simulink model "hwTarget"  (R2020b)
settings: Solver=VariableStepAuto  StartTime=0.0  StopTime=Ts  RelTol=1e-3
InitFcn:
  | evalin('base','pixelcontrolbus');
  | 
  | ROWS = 480;
  | COLS = 752;
  | 
  | OFFSET = 3;
  | imagesToRead = 20;
  | Ts = (imagesToRead + OFFSET) * 2;
  | 
  | inputNums = [1:imagesToRead];
  | 
  | MagThrL = 7;
  | MagThrS = 3;
  | SegMaxLength = 630;
  | 
  | NUM_OF_BITS = 32;
  | MSB = NUM_OF_BITS-1;
  | cap_1 = fixdt(0,NUM_OF_BITS,NUM_OF_BITS-1);
  | cap_2 = fixdt(0,NUM_OF_BITS,NUM_OF_BITS-2);
  | 
  | CORDIC_LUT_DT_1 = fixdt(1, NUM_OF_BITS, NUM_OF_BITS-2);
  | CORDIC_LUT_DT_2 = fixdt(1, NUM_OF_BITS, NUM_OF_BITS-1);
  | CORDIC_LUT_DT_3 = fixdt(1, NUM_OF_BITS, NUM_OF_BITS);
  | CORDIC_LUT_DT_4 = fixdt(1, NUM_OF_BITS, NUM_OF_BITS+1);
  | CORDIC_LUT_DT_5 = fixdt(1, NUM_OF_BITS, NUM_OF_BITS+1);
  | CORDIC_LUT_DT_6 = fixdt(1, NUM_OF_BITS, NUM_OF_BITS+2);
  | CORDIC_LUT_DT_7 = fixdt(1, NUM_OF_BITS, NUM_OF_BITS+3);
  | CORDIC_LUT_DT_8 = fixdt(1, NUM_OF_BITS, NUM_OF_BITS+4);
  | CORDIC_LUT_DT_9 = fixdt(1, NUM_OF_BITS, NUM_OF_BITS+5);
  | CORDIC_LUT_DT_10 = fixdt(1, NUM_OF_BITS, NUM_OF_BITS+6);
  | CORDIC_LUT_DT_11 = fixdt(1, NUM_OF_BITS, NUM_OF_BITS+7);
  | CORDIC_LUT_DT_12 = fixdt(1, NUM_OF_BITS, NUM_OF_BITS+8);
  | 
  | RGB_DT = fixdt(0, 24, 0);
  | GRAY_DT = fixdt(0, 8, 0);
  | THETA_DT = fixdt(1, 16, 13);
  | MAG_DT = fixdt(0, 16, 15);
  | KIRCH_DT = fixdt(0, 12, 0);
undefined symbols (not defined in the file or in its folder): bufferInit, bufferSize
libraries: hdlsllib x86, simulink x6, visionhdlstatistics x4, visionhdlio x2, visionhdlutilities x1
(part 3 of 3)

== system hwTarget/hwTarget/Kirsch Operation Northwest/Kirch Filter North-West/Kirch Filter/slicer ==
  note: 5 | 5 |-3
      | 5 | 0 |-3
      | -3 |-3 |-3
  data_in : Inport
  Delay{1..6} (6 alike) : Delay  DelayLength=1  InitialCondition=0
  Display : Display
  Display1 : Display
  Line buffer : Delay  DelayLength=COLS-2  InitialCondition=0
  Line buffer1 : Delay  DelayLength=COLS-2  InitialCondition=0
  Mux : Mux  Inputs=3
  Mux1 : Mux  Inputs=5
  Fives : Outport
  nThrees : Outport  Port=2
  wires:
  Delay4/1 -> Mux1/3, Line buffer/1
  data_in/1 -> Mux1/5, Delay1/1
  Delay1/1 -> Mux1/4, Delay4/1
  Delay3/1 -> Mux/2, Delay6/1
  Delay5/1 -> Line buffer1/1, Mux/3
  Line buffer/1 -> Mux1/2, Delay2/1
  Line buffer1/1 -> Delay3/1, Mux1/1
  Delay2/1 -> Delay5/1
  Mux/1 -> Display1/1, Fives/1
  Mux1/1 -> Display/1, nThrees/1
  Delay6/1 -> Mux/1

== system hwTarget/hwTarget/Kirsch Operation Southwest/Binarize/Subsystem/MagThrL ==
  mean : Inport
  stddev : Inport  Port=2
  dev_step : Inport  Port=3
  Add1 : Sum
  Product : Product
  thresh : Outport
  wires:
  stddev/1 -> Product/1
  mean/1 -> Add1/1
  dev_step/1 -> Product/2
  Product/1 -> Add1/2
  Add1/1 -> thresh/1

== system hwTarget/hwTarget/Kirsch Operation Southwest/Binarize/Subsystem/MagThrS ==
  mean : Inport
  stddev : Inport  Port=2
  dev_step : Inport  Port=3
  Add1 : Sum
  Product : Product
  thresh : Outport
  wires:
  stddev/1 -> Product/1
  mean/1 -> Add1/1
  dev_step/1 -> Product/2
  Product/1 -> Add1/2
  Add1/1 -> thresh/1

== system hwTarget/hwTarget/Kirsch Operation Southwest/Kirch Filter South-West/Subsystem/slicer ==
  note: -3 |-3 |-3
      | 5 | 0 |-3
      | 5 | 5 |-3
  data_in : Inport
  Delay{1..6} (6 alike) : Delay  DelayLength=1  InitialCondition=0
  Display : Display
  Display1 : Display
  Line buffer : Delay  DelayLength=COLS-2  InitialCondition=0
  Line buffer1 : Delay  DelayLength=COLS-2  InitialCondition=0
  Mux : Mux  Inputs=3
  Mux1 : Mux  Inputs=5
  Fives : Outport
  nThrees : Outport  Port=2
  wires:
  Delay4/1 -> Line buffer/1, Mux/2
  data_in/1 -> Mux1/5, Delay1/1
  Delay1/1 -> Mux/3, Delay4/1
  Delay3/1 -> Mux1/2, Delay6/1
  Delay5/1 -> Line buffer1/1, Mux/1
  Line buffer/1 -> Mux1/4, Delay2/1
  Line buffer1/1 -> Mux1/3, Delay3/1
  Delay2/1 -> Delay5/1
  Mux/1 -> Display1/1, Fives/1
  Mux1/1 -> Display/1, nThrees/1
  Delay6/1 -> Mux1/1

== system hwTarget/hwTarget/Kirsch Operation West/Binarize/Subsystem/MagThrL ==
  mean : Inport
  stddev : Inport  Port=2
  dev_step : Inport  Port=3
  Add1 : Sum
  Product : Product
  thresh : Outport
  wires:
  stddev/1 -> Product/1
  mean/1 -> Add1/1
  dev_step/1 -> Product/2
  Product/1 -> Add1/2
  Add1/1 -> thresh/1

== system hwTarget/hwTarget/Kirsch Operation West/Binarize/Subsystem/MagThrS ==
  mean : Inport
  stddev : Inport  Port=2
  dev_step : Inport  Port=3
  Add1 : Sum
  Product : Product
  thresh : Outport
  wires:
  stddev/1 -> Product/1
  mean/1 -> Add1/1
  dev_step/1 -> Product/2
  Product/1 -> Add1/2
  Add1/1 -> thresh/1

== system hwTarget/hwTarget/Kirsch Operation West/Kirch Filter West/Subsystem/slicer ==
  note: 5 |-3 |-3
      | 5 | 0 |-3
      | 5 |-3 |-3
  data_in : Inport
  Delay{1..6} (6 alike) : Delay  DelayLength=1  InitialCondition=0
  Display : Display
  Display1 : Display
  Line buffer : Delay  DelayLength=COLS-2  InitialCondition=0
  Line buffer1 : Delay  DelayLength=COLS-2  InitialCondition=0
  Mux : Mux  Inputs=3
  Mux1 : Mux  Inputs=5
  Fives : Outport
  nThrees : Outport  Port=2
  wires:
  Delay4/1 -> Mux/3, Line buffer/1
  data_in/1 -> Mux1/5, Delay1/1
  Delay1/1 -> Mux1/4, Delay4/1
  Delay3/1 -> Mux1/1, Delay6/1
  Delay5/1 -> Mux/2, Line buffer1/1
  Line buffer/1 -> Mux1/3, Delay2/1
  Line buffer1/1 -> Mux1/2, Delay3/1
  Delay2/1 -> Delay5/1
  Mux/1 -> Display1/1, Fives/1
  Mux1/1 -> Display/1, nThrees/1
  Delay6/1 -> Mux/1

== system hwTarget/hwTarget/Segmentation/North Segmentation/Enabled Subsystem1/Enabled Subsystem ==
  In1 : Inport
  Enable : EnablePort
  To Workspace7 : ToWorkspace  VariableName=officialResults  SaveFormat=Timeseries  SampleTime=-1
  wires:
  In1/1 -> To Workspace7/1

== system hwTarget/hwTarget/Segmentation/North Segmentation/Enabled Subsystem1/Subsystem ==
  u : Inport
  Bit Slice : hdlsllib/Logic and Bit Operations/Bit Slice  lidx=47  ridx=32
      settings: SourceProductBaseCode=SL
  Bit Slice1 : hdlsllib/Logic and Bit Operations/Bit Slice  lidx=31  ridx=16
      settings: SourceProductBaseCode=SL
  Bit Slice2 : hdlsllib/Logic and Bit Operations/Bit Slice  lidx=15  ridx=0
      settings: SourceProductBaseCode=SL
  x : Outport
  y : Outport  Port=2
  theta : Outport  Port=3
  wires:
  u/1 -> Bit Slice2/1, Bit Slice1/1, Bit Slice/1
  Bit Slice2/1 -> theta/1
  Bit Slice/1 -> x/1
  Bit Slice1/1 -> y/1

== system hwTarget/hwTarget/Segmentation/North Segmentation/Enabled Subsystem1/Subsystem1 ==
  u : Inport
  Bit Slice : hdlsllib/Logic and Bit Operations/Bit Slice  lidx=47  ridx=32
      settings: SourceProductBaseCode=SL
  Bit Slice1 : hdlsllib/Logic and Bit Operations/Bit Slice  lidx=31  ridx=16
      settings: SourceProductBaseCode=SL
  Bit Slice2 : hdlsllib/Logic and Bit Operations/Bit Slice  lidx=15  ridx=0
      settings: SourceProductBaseCode=SL
  x : Outport
  y : Outport  Port=2
  theta : Outport  Port=3
  wires:
  Bit Slice1/1 -> y/1
  Bit Slice/1 -> x/1
  Bit Slice2/1 -> theta/1
  u/1 -> Bit Slice/1, Bit Slice1/1, Bit Slice2/1

== system hwTarget/hwTarget/Segmentation/North Segmentation/Enabled Subsystem1/Subsystem2 ==
  u : Inport
  Bit Slice : hdlsllib/Logic and Bit Operations/Bit Slice  lidx=47  ridx=32
      settings: SourceProductBaseCode=SL
  Bit Slice1 : hdlsllib/Logic and Bit Operations/Bit Slice  lidx=31  ridx=16
      settings: SourceProductBaseCode=SL
  Bit Slice2 : hdlsllib/Logic and Bit Operations/Bit Slice  lidx=15  ridx=0
      settings: SourceProductBaseCode=SL
  x : Outport
  y : Outport  Port=2
  theta : Outport  Port=3
  wires:
  u/1 -> Bit Slice2/1, Bit Slice1/1, Bit Slice/1
  Bit Slice2/1 -> theta/1
  Bit Slice/1 -> x/1
  Bit Slice1/1 -> y/1

== system hwTarget/hwTarget/Segmentation/North Segmentation/Enabled Subsystem1/Subsystem3 ==
  u : Inport
  Bit Slice : hdlsllib/Logic and Bit Operations/Bit Slice  lidx=47  ridx=32
      settings: SourceProductBaseCode=SL
  Bit Slice1 : hdlsllib/Logic and Bit Operations/Bit Slice  lidx=31  ridx=16
      settings: SourceProductBaseCode=SL
  Bit Slice2 : hdlsllib/Logic and Bit Operations/Bit Slice  lidx=15  ridx=0
      settings: SourceProductBaseCode=SL
  x : Outport
  y : Outport  Port=2
  theta : Outport  Port=3
  wires:
  Bit Slice1/1 -> y/1
  Bit Slice/1 -> x/1
  Bit Slice2/1 -> theta/1
  u/1 -> Bit Slice/1, Bit Slice1/1, Bit Slice2/1

== system hwTarget/hwTarget/Segmentation/North Segmentation/minXReadSwitch/Subsystem1 ==
  reset : Inport
  Constant : Constant  OutDataTypeStr=fixdt(0,10,0)  SampleTime=-1
  Delay2 : Delay  DelayLength=1  InitialCondition=0  ExternalReset=Level
      settings: InputPortMap=u0,r5
  Sum : Sum  Inputs=|++  OutDataTypeStr=uint16
  counter : Outport
  wires:
  reset/1 -> Delay2/2
  Delay2/1 -> Sum/1
  Constant/1 -> Sum/2
  Sum/1 -> Delay2/1, counter/1  "blobID"

== system hwTarget/hwTarget/Segmentation/North Segmentation/minXReadSwitch1/Subsystem1 ==
  reset : Inport
  Constant : Constant  OutDataTypeStr=fixdt(0,10,0)  SampleTime=-1
  Delay2 : Delay  DelayLength=1  InitialCondition=0  ExternalReset=Level
      settings: InputPortMap=u0,r5
  Sum : Sum  Inputs=|++  OutDataTypeStr=uint16
  counter : Outport
  wires:
  reset/1 -> Delay2/2
  Delay2/1 -> Sum/1
  Constant/1 -> Sum/2
  Sum/1 -> Delay2/1, counter/1  "blobID"

== system hwTarget/hwTarget/Segmentation/North Segmentation/minXReadSwitch3/Subsystem1 ==
  reset : Inport
  Constant : Constant  OutDataTypeStr=fixdt(0,10,0)  SampleTime=-1
  Delay2 : Delay  DelayLength=1  InitialCondition=0  ExternalReset=Level
      settings: InputPortMap=u0,r5
  Sum : Sum  Inputs=|++  OutDataTypeStr=uint16
  counter : Outport
  wires:
  reset/1 -> Delay2/2
  Delay2/1 -> Sum/1
  Constant/1 -> Sum/2
  Sum/1 -> Delay2/1, counter/1  "blobID"

== system hwTarget/hwTarget/Segmentation/North Segmentation/minXSwitch4/Subsystem ==
  reset : Inport
  Constant : Constant  OutDataTypeStr=fixdt(0,10,0)  SampleTime=-1
  Delay2 : Delay  DelayLength=1  InitialCondition=0  ExternalReset=Level
      settings: InputPortMap=u0,r5
  Sum : Sum  Inputs=|++  OutDataTypeStr=uint16
  counter : Outport
  wires:
  Sum/1 -> counter/1, Delay2/1  "blobID"
  Constant/1 -> Sum/2
  Delay2/1 -> Sum/1
  reset/1 -> Delay2/2

== system hwTarget/hwTarget/Segmentation/North Segmentation/minXSwitch4/Subsystem1 ==
  reset : Inport
  Constant : Constant  OutDataTypeStr=fixdt(0,10,0)  SampleTime=-1
  Delay2 : Delay  DelayLength=1  InitialCondition=0  ExternalReset=Level
      settings: InputPortMap=u0,r5
  Sum : Sum  Inputs=|++  OutDataTypeStr=uint16
  counter : Outport
  wires:
  reset/1 -> Delay2/2
  Delay2/1 -> Sum/1
  Constant/1 -> Sum/2
  Sum/1 -> Delay2/1, counter/1  "blobID"

== system hwTarget/hwTarget/CordicAtan/CORDIC Algorithm/Iteration_10/X_Logic/zsign ==
  signof : Inport
  base : Inport  Port=2
  Bit Slice : hdlsllib/Logic and Bit Operations/Bit Slice  lidx=MSB  ridx=MSB
      settings: SourceProductBaseCode=SL
  Switch : Switch  Criteria=u2 > Threshold
  Unary Minus : UnaryMinus
  out : Outport
  wires:
  signof/1 -> Bit Slice/1
  Bit Slice/1 -> Switch/2
  base/1 -> Switch/3, Unary Minus/1
  Switch/1 -> out/1
  Unary Minus/1 -> Switch/1

== system hwTarget/hwTarget/CordicAtan/CORDIC Algorithm/Iteration_10/Y_Logic/n_zsign ==
  signof : Inport
  base : Inport  Port=2
  Bit Slice : hdlsllib/Logic and Bit Operations/Bit Slice  lidx=MSB  ridx=MSB
      settings: SourceProductBaseCode=SL
  Switch : Switch  Criteria=u2 > Threshold
  Unary Minus : UnaryMinus
  out : Outport
  wires:
  Bit Slice/1 -> Switch/2
  signof/1 -> Bit Slice/1
  base/1 -> Switch/1, Unary Minus/1
  Switch/1 -> out/1
  Unary Minus/1 -> Switch/3

== system hwTarget/hwTarget/CordicAtan/CORDIC Algorithm/Iteration_2/X_Logic/zsign1 ==
  signof : Inport
  base : Inport  Port=2
  Bit Slice : hdlsllib/Logic and Bit Operations/Bit Slice  lidx=MSB  ridx=MSB
      settings: SourceProductBaseCode=SL
  Switch : Switch  Criteria=u2 > Threshold
  Unary Minus : UnaryMinus
  out : Outport
  wires:
  signof/1 -> Bit Slice/1
  Bit Slice/1 -> Switch/2
  base/1 -> Switch/3, Unary Minus/1
  Switch/1 -> out/1
  Unary Minus/1 -> Switch/1

== system hwTarget/hwTarget/CordicAtan/CORDIC Algorithm/Iteration_2/Y_Logic/n_zsign ==
  signof : Inport
  base : Inport  Port=2
  Bit Slice : hdlsllib/Logic and Bit Operations/Bit Slice  lidx=MSB  ridx=MSB
      settings: SourceProductBaseCode=SL
  Switch : Switch  Criteria=u2 > Threshold
  Unary Minus : UnaryMinus
  out : Outport
  wires:
  Bit Slice/1 -> Switch/2
  signof/1 -> Bit Slice/1
  base/1 -> Switch/1, Unary Minus/1
  Switch/1 -> out/1
  Unary Minus/1 -> Switch/3

== system hwTarget/hwTarget/CordicAtan/CORDIC Algorithm/Iteration_3/X_Logic/zsign ==
  signof : Inport
  base : Inport  Port=2
  Bit Slice : hdlsllib/Logic and Bit Operations/Bit Slice  lidx=MSB  ridx=MSB
      settings: SourceProductBaseCode=SL
  Switch : Switch  Criteria=u2 > Threshold
  Unary Minus : UnaryMinus
  out : Outport
  wires:
  signof/1 -> Bit Slice/1
  Bit Slice/1 -> Switch/2
  base/1 -> Switch/3, Unary Minus/1
  Switch/1 -> out/1
  Unary Minus/1 -> Switch/1

== system hwTarget/hwTarget/CordicAtan/CORDIC Algorithm/Iteration_3/Y_Logic/n_zsign ==
  signof : Inport
  base : Inport  Port=2
  Bit Slice : hdlsllib/Logic and Bit Operations/Bit Slice  lidx=MSB  ridx=MSB
      settings: SourceProductBaseCode=SL
  Switch : Switch  Criteria=u2 > Threshold
  Unary Minus : UnaryMinus
  out : Outport
  wires:
  Bit Slice/1 -> Switch/2
  signof/1 -> Bit Slice/1
  base/1 -> Switch/1, Unary Minus/1
  Switch/1 -> out/1
  Unary Minus/1 -> Switch/3

== system hwTarget/hwTarget/CordicAtan/CORDIC Algorithm/Iteration_4/X_Logic/zsign ==
  signof : Inport
  base : Inport  Port=2
  Bit Slice : hdlsllib/Logic and Bit Operations/Bit Slice  lidx=MSB  ridx=MSB
      settings: SourceProductBaseCode=SL
  Switch : Switch  Criteria=u2 > Threshold
  Unary Minus : UnaryMinus
  out : Outport
  wires:
  signof/1 -> Bit Slice/1
  Bit Slice/1 -> Switch/2
  base/1 -> Switch/3, Unary Minus/1
  Switch/1 -> out/1
  Unary Minus/1 -> Switch/1

== system hwTarget/hwTarget/CordicAtan/CORDIC Algorithm/Iteration_4/Y_Logic/n_zsign ==
  signof : Inport
  base : Inport  Port=2
  Bit Slice : hdlsllib/Logic and Bit Operations/Bit Slice  lidx=MSB  ridx=MSB
      settings: SourceProductBaseCode=SL
  Switch : Switch  Criteria=u2 > Threshold
  Unary Minus : UnaryMinus
  out : Outport
  wires:
  Bit Slice/1 -> Switch/2
  signof/1 -> Bit Slice/1
  base/1 -> Switch/1, Unary Minus/1
  Switch/1 -> out/1
  Unary Minus/1 -> Switch/3

== system hwTarget/hwTarget/CordicAtan/CORDIC Algorithm/Iteration_5/X_Logic/zsign ==
  signof : Inport
  base : Inport  Port=2
  Bit Slice : hdlsllib/Logic and Bit Operations/Bit Slice  lidx=MSB  ridx=MSB
      settings: SourceProductBaseCode=SL
  Switch : Switch  Criteria=u2 > Threshold
  Unary Minus : UnaryMinus
  out : Outport
  wires:
  signof/1 -> Bit Slice/1
  Bit Slice/1 -> Switch/2
  base/1 -> Switch/3, Unary Minus/1
  Switch/1 -> out/1
  Unary Minus/1 -> Switch/1

== system hwTarget/hwTarget/CordicAtan/CORDIC Algorithm/Iteration_5/Y_Logic/n_zsign ==
  signof : Inport
  base : Inport  Port=2
  Bit Slice : hdlsllib/Logic and Bit Operations/Bit Slice  lidx=MSB  ridx=MSB
      settings: SourceProductBaseCode=SL
  Switch : Switch  Criteria=u2 > Threshold
  Unary Minus : UnaryMinus
  out : Outport
  wires:
  Bit Slice/1 -> Switch/2
  signof/1 -> Bit Slice/1
  base/1 -> Switch/1, Unary Minus/1
  Switch/1 -> out/1
  Unary Minus/1 -> Switch/3

== system hwTarget/hwTarget/CordicAtan/CORDIC Algorithm/Iteration_6/X_Logic/zsign ==
  signof : Inport
  base : Inport  Port=2
  Bit Slice : hdlsllib/Logic and Bit Operations/Bit Slice  lidx=MSB  ridx=MSB
      settings: SourceProductBaseCode=SL
  Switch : Switch  Criteria=u2 > Threshold
  Unary Minus : UnaryMinus
  out : Outport
  wires:
  signof/1 -> Bit Slice/1
  Bit Slice/1 -> Switch/2
  base/1 -> Switch/3, Unary Minus/1
  Switch/1 -> out/1
  Unary Minus/1 -> Switch/1

== system hwTarget/hwTarget/CordicAtan/CORDIC Algorithm/Iteration_6/Y_Logic/n_zsign ==
  signof : Inport
  base : Inport  Port=2
  Bit Slice : hdlsllib/Logic and Bit Operations/Bit Slice  lidx=MSB  ridx=MSB
      settings: SourceProductBaseCode=SL
  Switch : Switch  Criteria=u2 > Threshold
  Unary Minus : UnaryMinus
  out : Outport
  wires:
  Bit Slice/1 -> Switch/2
  signof/1 -> Bit Slice/1
  base/1 -> Switch/1, Unary Minus/1
  Switch/1 -> out/1
  Unary Minus/1 -> Switch/3

== system hwTarget/hwTarget/CordicAtan/CORDIC Algorithm/Iteration_7/X_Logic/zsign ==
  signof : Inport
  base : Inport  Port=2
  Bit Slice : hdlsllib/Logic and Bit Operations/Bit Slice  lidx=MSB  ridx=MSB
      settings: SourceProductBaseCode=SL
  Switch : Switch  Criteria=u2 > Threshold
  Unary Minus : UnaryMinus
  out : Outport
  wires:
  signof/1 -> Bit Slice/1
  Bit Slice/1 -> Switch/2
  base/1 -> Switch/3, Unary Minus/1
  Switch/1 -> out/1
  Unary Minus/1 -> Switch/1

== system hwTarget/hwTarget/CordicAtan/CORDIC Algorithm/Iteration_7/Y_Logic/n_zsign ==
  signof : Inport
  base : Inport  Port=2
  Bit Slice : hdlsllib/Logic and Bit Operations/Bit Slice  lidx=MSB  ridx=MSB
      settings: SourceProductBaseCode=SL
  Switch : Switch  Criteria=u2 > Threshold
  Unary Minus : UnaryMinus
  out : Outport
  wires:
  Bit Slice/1 -> Switch/2
  signof/1 -> Bit Slice/1
  base/1 -> Switch/1, Unary Minus/1
  Switch/1 -> out/1
  Unary Minus/1 -> Switch/3

== system hwTarget/hwTarget/CordicAtan/CORDIC Algorithm/Iteration_8/X_Logic/zsign ==
  signof : Inport
  base : Inport  Port=2
  Bit Slice : hdlsllib/Logic and Bit Operations/Bit Slice  lidx=MSB  ridx=MSB
      settings: SourceProductBaseCode=SL
  Switch : Switch  Criteria=u2 > Threshold
  Unary Minus : UnaryMinus
  out : Outport
  wires:
  signof/1 -> Bit Slice/1
  Bit Slice/1 -> Switch/2
  base/1 -> Switch/3, Unary Minus/1
  Switch/1 -> out/1
  Unary Minus/1 -> Switch/1

== system hwTarget/hwTarget/CordicAtan/CORDIC Algorithm/Iteration_8/Y_Logic/n_zsign ==
  signof : Inport
  base : Inport  Port=2
  Bit Slice : hdlsllib/Logic and Bit Operations/Bit Slice  lidx=MSB  ridx=MSB
      settings: SourceProductBaseCode=SL
  Switch : Switch  Criteria=u2 > Threshold
  Unary Minus : UnaryMinus
  out : Outport
  wires:
  Bit Slice/1 -> Switch/2
  signof/1 -> Bit Slice/1
  base/1 -> Switch/1, Unary Minus/1
  Switch/1 -> out/1
  Unary Minus/1 -> Switch/3

== system hwTarget/hwTarget/CordicAtan/CORDIC Algorithm/Iteration_9/X_Logic/zsign ==
  signof : Inport
  base : Inport  Port=2
  Bit Slice : hdlsllib/Logic and Bit Operations/Bit Slice  lidx=MSB  ridx=MSB
      settings: SourceProductBaseCode=SL
  Switch : Switch  Criteria=u2 > Threshold
  Unary Minus : UnaryMinus
  out : Outport
  wires:
  signof/1 -> Bit Slice/1
  Bit Slice/1 -> Switch/2
  base/1 -> Switch/3, Unary Minus/1
  Switch/1 -> out/1
  Unary Minus/1 -> Switch/1

== system hwTarget/hwTarget/CordicAtan/CORDIC Algorithm/Iteration_9/Y_Logic/n_zsign ==
  signof : Inport
  base : Inport  Port=2
  Bit Slice : hdlsllib/Logic and Bit Operations/Bit Slice  lidx=MSB  ridx=MSB
      settings: SourceProductBaseCode=SL
  Switch : Switch  Criteria=u2 > Threshold
  Unary Minus : UnaryMinus
  out : Outport
  wires:
  Bit Slice/1 -> Switch/2
  signof/1 -> Bit Slice/1
  base/1 -> Switch/1, Unary Minus/1
  Switch/1 -> out/1
  Unary Minus/1 -> Switch/3

== matlab function hwTarget/Segmentation/North Segmentation/Enabled Subsystem/MATLAB Function ==
  data: left input uint16; pixel input boolean; x input uint16; assignment output uint16; y input uint16; theta input uint16; maxXAboveX input uint16; maxXAboveY input uint16; maxXAboveT input uint16; minXLeftX input uint16; minXLeftY input uint16; above input uint16; maxXLeftX input uint16; merger_addr output uint16; merger_data output uint16; minX_addr output uint16; minX_data output uint16; maxX_addr output uint16; maxX_data output uint16; minY_addr output uint16; minY_data output uint16; maxY_addr output uint16; maxY_data output uint16; merger_we output uint16; blobIDin input uint16; blobIDout output uint16 size=1; frameNum input; frame_end input
function [assignment,merger_addr,merger_data,minX_addr,minX_data,maxX_addr,maxX_data,minY_addr,minY_data,maxY_addr,maxY_data,merger_we,blobIDout] = fcn(left,pixel,x,y,theta,maxXAboveX,maxXAboveY,maxXAboveT,minXLeftX,minXLeftY,above,maxXLeftX,blobIDin,frameNum,frame_end)
    assignment = uint16(0);
    blobIDout = blobIDin;
    merger_we = uint16(0);
    merger_addr = uint16(0);
    merger_data = uint16(0);
    minX_addr = uint16(0);
    minX_data = [uint16(0) ;uint16(0);uint16(0)];
    maxX_addr = uint16(0);
    maxX_data = [uint16(0) ;uint16(0);uint16(0)];
    minY_addr = uint16(0);
    minY_data = [uint16(0) ;uint16(0);uint16(0)];
    maxY_addr = uint16(0);
    maxY_data = [uint16(0) ;uint16(0);uint16(0)];
        
    if (frameNum == 2)
        
        if (x == 98)
            if (y == 22)
                z =1;
            end
        end
                
            
        if (x == 1)
            left = uint16(0);
        end

        if (pixel == 0)
            assignment = uint16(0);
        else
            if ((left ~= 0) && (above ~= 0))
                merger_we = uint16(1);
                % merger
                if (left < above)
                    assignment = left;
                    
                    %%%%%%%%%%%%%%%%%%%%%%%%%%%%%%%%%
                    %mergerLookup(above) = left;
                    %%%%%%%%%%%%%%%%%%%%%%%%%%%%%%%%%
                    merger_addr = above;
                    merger_data = left;
                    
                    %%%%%%%%%%%%%%%%%%%%%%%%%%%%%%%%%%%%%
                    %maxX(left,:) = maxX(above,:);
                    %maxX(left,3) = theta(counter);
                    %%%%%%%%%%%%%%%%%%%%%%%%%%%%%%%%%%%%%
                    maxX_addr = left;
                    maxX_data = [maxXAboveX; maxXAboveY; theta];
                    
                elseif (above < left)
                    assignment = above;
                    
                    %%%%%%%%%%%%%%%%%%%%%%%%%%%%%%%%%%%%%
                    %mergerLookup(left) = above;
                    %%%%%%%%%%%%%%%%%%%%%%%%%%%%%%%%%%%%%
                    merger_addr = left;
                    merger_data = above;
                    
                    %%%%%%%%%%%%%%%%%%%%%%%%%%%%%%%%%%%%%
                    %minX(above,:) = minX(left,:);
                    %maxX(above,3) = theta(counter);
                    %%%%%%%%%%%%%%%%%%%%%%%%%%%%%%%%%%%%%
                    minX_addr = above;
                    minX_data = [minXLeftX; minXLeftY ;theta];
                    % TODO: the above line will not work when there is only
                    % a single bit to the left and then there is an
                    % instantateous merger.  The left pixels data does not
                    % have time to be written to the bram and be read out
                    % before it is needed.  As long ast here are two pixels
                    % to the left before the merger this works fine.
                else
                    %%%%%%%%%%%%%%%%%%%%%%%%%%%%%%%%%%%%%
                    %maxX(left,:) = maxX(above,:);
                    %%%%%%%%%%%%%%%%%%%%%%%%%%%%%%%%%%%%%%
                    maxX_addr = left;
                    maxX_data = [maxXAboveX; maxXAboveY; maxXAboveT];
                end
            elseif ((left ~= 0) && (above == 0))
                % take left id
                assignment = left;
                
                % only update the maxX point
                %%%%%%%%%%%%%%%%%%%%%%%%%%%%%
                %if (x > maxX(left,1))
                %   maxX(left,:) = [x,y,theta(counter),1];
                %end
                %%%%%%%%%%%%%%%%%%%%%%%%%%%%%
                if (x > maxXLeftX)
                    maxX_addr = left;
                    maxX_data = [x ;y; theta];
                end
                
            elseif ((left == 0) && (above ~= 0))
                % take above id
                assignment = above;
                
                % only update the maxY point
                %%%%%%%%%%%%%%%%%%%%%%%%%%%%%%%%%%%%%%%%%%%%
                % maxY(above,:) = [x,y,theta(counter),1];
                %%%%%%%%%%%%%%%%%%%%%%%%%%%%%%%%%%%%%%%%%%%%
                maxY_addr = above;
                maxY_data = [x ;y ;theta];
            else
                % new ID
                %%%%%%%%%%%%%%%%%%%%%%%%%%%%%
                %blobID = blobID + 1;
                %%%%%%%%%%%%%%%%%%%%%%%%%%%%%
                blobIDout = blobIDin + uint16(1);
                assignment = blobIDin;
                    
                % load in all bram entries and mark as valid
                %%%%%%%%%%%%%%%%%%%%%%%%%%%%%%%%%%%%%%%%%%%%
                %minX(blobID,:) = [x,y,theta(counter),1];
                %maxX(blobID,:) = [x,y,theta(counter),1];
                %minY(blobID,:) = [x,y,theta(counter),1];
                %maxY(blobID,:) = [x,y,theta(counter),1];
                %%%%%%%%%%%%%%%%%%%%%%%%%%%%%%%%%%%%%%%%%%%%
                minX_addr = blobIDin;
                maxX_addr = blobIDin;
                minY_addr = blobIDin;
                maxY_addr = blobIDin;
                minX_data = [x ;y; theta];
                maxX_data = [x ;y; theta];
                minY_data = [x ;y; theta];
                maxY_data = [x ;y; theta];
            end
            
            if (frame_end == 1)
                    blobIDout = uint16(1);
            end
        end
    end
end

== matlab function hwTarget/Image Loader/MATLAB Function ==
  data: images output; simTime input
function images = load_images(simTime)

coder.extrinsic('fullfile');

local_path = "../../matlab/pics/data/";

persistent imageNum

if isempty(imageNum)
    imageNum = 1;
end

images = uint8(zeros(480,752,3));
file = sprintf("input%d.bmp", int16(imageNum));
path = fullfile(local_path, file);
images = uint8(imread(path));
if simTime > 2
    imageNum = imageNum + 1;
end

== matlab function hwTarget/Segmentation/North Segmentation/Enabled Subsystem1/MATLAB Function ==
  data: minXx input; x1 output uint16; minXy input; minXtheta input; maxXx input; maxXy input; maxXtheta input; minYx input; minYy input; minYtheta input; maxYx input; maxYy input; maxYtheta input; merger input; index input; y1 output uint16; x2 output uint16; y2 output uint16; theta output uint16; lineThreshold input; w_addr_in input; we output; w_addr_out output
function [x1,y1,x2,y2,theta,we,w_addr_out] = fcn(minXx,minXy,minXtheta,maxXx,maxXy,maxXtheta,minYx,minYy,minYtheta,maxYx,maxYy,maxYtheta,merger,index,lineThreshold,w_addr_in)

theta = minXtheta;
we = uint16(0);
w_addr_out = w_addr_in;
flag = uint16(0);

if (merger == index)
   % have a valid segment, so find the longest line
   line1 = uint16(abs(int16(minXx)-int16(maxXx)) + abs(int16(minXy)-int16(maxXy)));
   line2 = uint16(abs(int16(minXx)-int16(minYx)) + abs(int16(minXy)-int16(minYy)));
   line3 = uint16(abs(int16(minXx)-int16(maxYx)) + abs(int16(minXy)-int16(maxYy)));
   line4 = uint16(abs(int16(maxXx)-int16(minYx)) + abs(int16(maxXy)-int16(minYy)));
   line5 = uint16(abs(int16(maxXx)-int16(maxYx)) + abs(int16(maxXy)-int16(maxYy)));
   line6 = uint16(abs(int16(minYx)-int16(maxYx)) + abs(int16(minYy)-int16(maxYy)));
   
   x1 = uint16(0);
   y1 = uint16(0);
   x2 = uint16(0);
   y2 = uint16(0);
   maxLine = lineThreshold;
   
   if(line1>maxLine)
       x1 = minXx;
       y1 = minXy;
       x2 = maxXx;
       y2 = maxXy;
       maxLine = line1;
       flag = uint16(1);
   end
   
   if(line2>maxLine)
       x1 = minXx;
       y1 = minXy;
       x2 = minYx;
       y2 = minYy;
       maxLine = line2;
       flag = uint16(1);
   end
  
   if(line3>maxLine)
       x1 = minXx;
       y1 = minXy;
       x2 = maxYx;
       y2 = maxYy;
       maxLine = line3;
       flag = uint16(1);
   end 
   
   if(line4>maxLine)
       x1 = maxXx;
       y1 = maxXy;
       x2 = minYx;
       y2 = minYy;
       maxLine = line4;
       flag = uint16(1);
   end 
   
   if(line5>maxLine)
       x1 = maxXx;
       y1 = maxXy;
       x2 = maxYx;
       y2 = maxYy;
       maxLine = line5;
       flag = uint16(1);
   end
   
   if(line6>maxLine)
       x1 = minYx;
       y1 = minYy;
       x2 = maxYx;
       y2 = maxYy;
       maxLine = line6;
       flag = uint16(1);
   end 
   
   if(flag == 1)
        we = uint16(1);
        w_addr_out = w_addr_in + 1;
   end
   
else
   x1 = uint16(0);
   y1 = uint16(0);
   x2 = uint16(0);
   y2 = uint16(0);
   theta = uint16(0);
end
